simulink model "EPT"  (R2019b)
settings: Solver=FixedStepDiscrete  StartTime=0.0  StopTime=5  FixedStep=0.005  RelTol=1e-3  EnableMultiTasking=on
PreLoadFcn:
  | try, model_open; catch, disp('Error occurred while executing model pre-load callback: model_open.m'); disp('Please assure that the MATLAB working directory is set to the model directory before opening.'); end
InitFcn:
  | try, model_open; catch, end
undefined symbols (not defined in the file or in its folder): Bridge, GCM, H, ln, raptor_get_param_eval, raptor_get_safe_string, raptor_xcp_function
libraries: Raptor_lib x2810, simulink x374, hdlsllib x19
(part 15 of 45)

== system EPT/Foreground_TimeBase_5ms/CAN/CAN2_exec/BCU vs ITRI//ARTC/Remote DAG2-5E1 ==
  Enable : EnablePort
  Trigger : TriggerPort  VariantControl=Variant  PortDimensions=1
  Data Type Conversion{1..4} (4 alike) : DataTypeConversion
  Fcn1 : Fcn  Expr=(u(1)-2)/0.01
  Fcn2 : Fcn  Expr=(u(1)-2)/0.01
  Fcn3 : Fcn  Expr=(u(1)+40)/0.5
  Fcn4 : Fcn  Expr=(u(1)+40)/0.5
  raptor_can_txmsg : Raptor_lib/CAN/raptor_can_txmsg  canDefinition=struct('dbcFile', 'BCUvsRMDA_CMU.dbc','message', 'RemoteDAG_5E1','comment', '','signals', {{'CMU1_Ibp','CMU1_Tcell_Max','CMU1_Tcell_Min','CMU1_Vbp','CMU1_Vcell_Max','CMU1_Vcell_Min'}},'enabled', [ 1 1 1 1 1 1;],'canBus', '''CAN2''','messageID', [ 1505;],'idMask', [ 536870911;],'payloadMask', [],'payloadValue', [],'period', [ 0;],'mailbox', '','queueSize', [ 1;],'label', [ 0;],'ver', [ 2;],'showID', [ 0;],'showRaw', [ 0;],'fill', [ 0;],'editID', [ 0;],'signalOrder', [ 1;])  canBus='CAN2'  queueSize=1  payloadMask=[]  payloadValue=[]  period=0  showID=0  label=0  idMask=hex2dec('1FFFFFFF')  fill=0  id=1505  showRaw=0  signalOrder=1  signalInfo={{struct('Name', 'CMU1_Ibp','Startbit', [ 0;],'SignalSize', [ 16;],'ByteOrder', 'BigEndian','ValueType', 'UNSIGNED','Class', 'uint16','Signed', [ 0;],'Factor', [ 0.02;],'Offset', [ -500;],'Min', [ 0;],'Max', [ 0;],'Units', '','Comment', '','StartBit', [ 8;]),struct('Name', 'CMU1_Vbp','Startbit', [ 0;],'SignalSize', [ 16;],'ByteOrder', 'BigEndian','ValueType', 'UNSIGNED','Class', 'uint16','Signed', [ 0;],'Factor', [ 0.01;],'Offset', [ 0;],'Min', [ 0;],'Max', [ 0;],'Units', '','Comment', '','StartBit', [ 24;]),struct('Name', 'CMU1_Vcell_Max','Startbit', [ 0;],'SignalSize', [ 8;],'ByteOrder', 'BigEndian','ValueType', 'UNSIGNED','Class', 'uint8','Signed', [ 0;],'Factor', [ 1;],'Offset', [ 0;],'Min', [ 0;],'Max', [ 0;],'Units', '','Comment', '','StartBit', [ 32;]),struct('Name', 'CMU1_Vcell_Min','Startbit', [ 0;],'SignalSize', [ 8;],'ByteOrder', 'BigEndian','ValueType', 'UNSIGNED','Class', 'uint8','Signed', [ 0;],'Factor', [ 1;],'Offset', [ 0;],'Min', [ 0;],'Max', [ 0;],'Units', '','Comment', '','StartBit', [ 40;]),struct('Name', 'CMU1_Tcell_Max','Startbit', [ 0;],'SignalSize', [ 8;],'ByteOrder', 'BigEndian','ValueType', 'UNSIGNED','Class', 'uint8','Signed', [ 0;],'Factor', [ 1;],'Offset', [ 0;],'Min', [ 0;],'Max', [ 0;],'Units', '','Comment', '','StartBit', [ 48;]),struct('Name', 'CMU1_Tcell_Min','Startbit', [ 0;],'SignalSize', [ 8;],'ByteOrder', 'BigEndian','ValueType', 'UNSIGNED','Class', 'uint8','Signed', [ 0;],'Factor', [ 1;],'Offset', [ 0;],'Min', [ 0;],'Max', [ 0;],'Units', '','Comment', '','StartBit', [ 56;])}}
      settings: SourceProductName=Raptor
  raptor_data_read : Raptor_lib/Data Storage/raptor_data_read  dataName='CMU1_CELL_VOLT_MAX'  dataShape=Scalar  idxSource=Input  idxRow=1  idxCol=1
      settings: SourceProductName=Raptor
  raptor_data_read1 : Raptor_lib/Data Storage/raptor_data_read  dataName='CMU1_CELL_VOLT_MIN'  dataShape=Scalar  idxSource=Input  idxRow=1  idxCol=1
      settings: SourceProductName=Raptor
  raptor_data_read2 : Raptor_lib/Data Storage/raptor_data_read  dataName='CMU1_CELL_TEMP_MIN'  dataShape=Scalar  idxSource=Input  idxRow=1  idxCol=1
      settings: SourceProductName=Raptor
  raptor_data_read3 : Raptor_lib/Data Storage/raptor_data_read  dataName='CMU1_BATT_CURR'  dataShape=Scalar  idxSource=Input  idxRow=1  idxCol=1
      settings: SourceProductName=Raptor
  raptor_data_read4 : Raptor_lib/Data Storage/raptor_data_read  dataName='CMU1_BATT_VOLT'  dataShape=Scalar  idxSource=Input  idxRow=1  idxCol=1
      settings: SourceProductName=Raptor
  raptor_data_read5 : Raptor_lib/Data Storage/raptor_data_read  dataName='CMU1_CELL_TEMP_MAX'  dataShape=Scalar  idxSource=Input  idxRow=1  idxCol=1
      settings: SourceProductName=Raptor
  wires:
  Fcn4/1 -> Data Type Conversion3/1
  Data Type Conversion3/1 -> raptor_can_txmsg/3
  raptor_data_read2/1 -> Fcn4/1
  raptor_data_read5/1 -> Fcn3/1
  Data Type Conversion2/1 -> raptor_can_txmsg/2
  Fcn3/1 -> Data Type Conversion2/1
  Data Type Conversion1/1 -> raptor_can_txmsg/5
  Data Type Conversion4/1 -> raptor_can_txmsg/6
  Fcn1/1 -> Data Type Conversion4/1
  Fcn2/1 -> Data Type Conversion1/1
  raptor_data_read4/1 -> raptor_can_txmsg/4
  raptor_data_read3/1 -> raptor_can_txmsg/1
  raptor_data_read1/1 -> Fcn1/1
  raptor_data_read/1 -> Fcn2/1

== system EPT/Foreground_TimeBase_5ms/CAN/CAN2_exec/BCU vs ITRI//ARTC/Remote DAG2-5E2 ==
  Enable : EnablePort
  Trigger : TriggerPort  VariantControl=Variant  PortDimensions=1
  Data Type Conversion{1..8} (8 alike) : DataTypeConversion
  Fcn{,1..7} (8 alike) : Fcn  Expr=(u(1)-2)/0.01
  raptor_can_txmsg : Raptor_lib/CAN/raptor_can_txmsg  canDefinition=struct('dbcFile', 'BCUvsRMDA_CMU.dbc','message', 'RemoteDAG_5E2','comment', '','signals', {{'CMU1_Vcell_V01','CMU1_Vcell_V02','CMU1_Vcell_V03','CMU1_Vcell_V04','CMU1_Vcell_V05','CMU1_Vcell_V06','CMU1_Vcell_V07','CMU1_Vcell_V08'}},'enabled', [ 1 1 1 1 1 1 1 1;],'canBus', '''CAN2''','messageID', [ 1506;],'idMask', [ 536870911;],'payloadMask', [],'payloadValue', [],'period', [ 0;],'mailbox', '','queueSize', [ 1;],'label', [ 0;],'ver', [ 2;],'showID', [ 0;],'showRaw', [ 0;],'fill', [ 0;],'editID', [ 0;],'signalOrder', [ 1;])  canBus='CAN2'  queueSize=1  payloadMask=[]  payloadValue=[]  period=0  showID=0  label=0  idMask=hex2dec('1FFFFFFF')  fill=0  id=1506  showRaw=0  signalOrder=1  signalInfo={{struct('Name', 'CMU1_Vcell_V01','Startbit', [ 0;],'SignalSize', [ 8;],'ByteOrder', 'BigEndian','ValueType', 'UNSIGNED','Class', 'uint8','Signed', [ 0;],'Factor', [ 1;],'Offset', [ 0;],'Min', [ 0;],'Max', [ 0;],'Units', '','Comment', '','StartBit', [ 0;]),struct('Name', 'CMU1_Vcell_V02','Startbit', [ 0;],'SignalSize', [ 8;],'ByteOrder', 'BigEndian','ValueType', 'UNSIGNED','Class', 'uint8','Signed', [ 0;],'Factor', [ 1;],'Offset', [ 0;],'Min', [ 0;],'Max', [ 0;],'Units', '','Comment', '','StartBit', [ 8;]),struct('Name', 'CMU1_Vcell_V03','Startbit', [ 0;],'SignalSize', [ 8;],'ByteOrder', 'BigEndian','ValueType', 'UNSIGNED','Class', 'uint8','Signed', [ 0;],'Factor', [ 1;],'Offset', [ 0;],'Min', [ 0;],'Max', [ 0;],'Units', '','Comment', '','StartBit', [ 16;]),struct('Name', 'CMU1_Vcell_V04','Startbit', [ 0;],'SignalSize', [ 8;],'ByteOrder', 'BigEndian','ValueType', 'UNSIGNED','Class', 'uint8','Signed', [ 0;],'Factor', [ 1;],'Offset', [ 0;],'Min', [ 0;],'Max', [ 0;],'Units', '','Comment', '','StartBit', [ 24;]),struct('Name', 'CMU1_Vcell_V05','Startbit', [ 0;],'SignalSize', [ 8;],'ByteOrder', 'BigEndian','ValueType', 'UNSIGNED','Class', 'uint8','Signed', [ 0;],'Factor', [ 1;],'Offset', [ 0;],'Min', [ 0;],'Max', [ 0;],'Units', '','Comment', '','StartBit', [ 32;]),struct('Name', 'CMU1_Vcell_V06','Startbit', [ 0;],'SignalSize', [ 8;],'ByteOrder', 'BigEndian','ValueType', 'UNSIGNED','Class', 'uint8','Signed', [ 0;],'Factor', [ 1;],'Offset', [ 0;],'Min', [ 0;],'Max', [ 0;],'Units', '','Comment', '','StartBit', [ 40;]),struct('Name', 'CMU1_Vcell_V07','Startbit', [ 0;],'SignalSize', [ 8;],'ByteOrder', 'BigEndian','ValueType', 'UNSIGNED','Class', 'uint8','Signed', [ 0;],'Factor', [ 1;],'Offset', [ 0;],'Min', [ 0;],'Max', [ 0;],'Units', '','Comment', '','StartBit', [ 48;]),struct('Name', 'CMU1_Vcell_V08','Startbit', [ 0;],'SignalSize', [ 8;],'ByteOrder', 'BigEndian','ValueType', 'UNSIGNED','Class', 'uint8','Signed', [ 0;],'Factor', [ 1;],'Offset', [ 0;],'Min', [ 0;],'Max', [ 0;],'Units', '','Comment', '','StartBit', [ 56;])}}
      settings: SourceProductName=Raptor
  raptor_data_read1 : Raptor_lib/Data Storage/raptor_data_read  dataName='CMU1_CELL02_VOLT'  dataShape=Scalar  idxSource=Input  idxRow=1  idxCol=1
      settings: SourceProductName=Raptor
  raptor_data_read2 : Raptor_lib/Data Storage/raptor_data_read  dataName='CMU1_CELL03_VOLT'  dataShape=Scalar  idxSource=Input  idxRow=1  idxCol=1
      settings: SourceProductName=Raptor
  raptor_data_read3 : Raptor_lib/Data Storage/raptor_data_read  dataName='CMU1_CELL01_VOLT'  dataShape=Scalar  idxSource=Input  idxRow=1  idxCol=1
      settings: SourceProductName=Raptor
  raptor_data_read4 : Raptor_lib/Data Storage/raptor_data_read  dataName='CMU1_CELL04_VOLT'  dataShape=Scalar  idxSource=Input  idxRow=1  idxCol=1
      settings: SourceProductName=Raptor
  raptor_data_read5 : Raptor_lib/Data Storage/raptor_data_read  dataName='CMU1_CELL05_VOLT'  dataShape=Scalar  idxSource=Input  idxRow=1  idxCol=1
      settings: SourceProductName=Raptor
  raptor_data_read6 : Raptor_lib/Data Storage/raptor_data_read  dataName='CMU1_CELL06_VOLT'  dataShape=Scalar  idxSource=Input  idxRow=1  idxCol=1
      settings: SourceProductName=Raptor
  raptor_data_read7 : Raptor_lib/Data Storage/raptor_data_read  dataName='CMU1_CELL07_VOLT'  dataShape=Scalar  idxSource=Input  idxRow=1  idxCol=1
      settings: SourceProductName=Raptor
  raptor_data_read8 : Raptor_lib/Data Storage/raptor_data_read  dataName='CMU1_CELL08_VOLT'  dataShape=Scalar  idxSource=Input  idxRow=1  idxCol=1
      settings: SourceProductName=Raptor
  wires:
  raptor_data_read7/1 -> Fcn6/1
  raptor_data_read6/1 -> Fcn5/1
  raptor_data_read5/1 -> Fcn4/1
  raptor_data_read4/1 -> Fcn3/1
  raptor_data_read2/1 -> Fcn2/1
  raptor_data_read3/1 -> Fcn/1
  Data Type Conversion4/1 -> raptor_can_txmsg/1
  Fcn1/1 -> Data Type Conversion8/1
  Fcn2/1 -> Data Type Conversion7/1
  Fcn7/1 -> Data Type Conversion3/1
  Data Type Conversion2/1 -> raptor_can_txmsg/7
  Data Type Conversion8/1 -> raptor_can_txmsg/2
  Data Type Conversion1/1 -> raptor_can_txmsg/6
  Data Type Conversion5/1 -> raptor_can_txmsg/5
  Data Type Conversion6/1 -> raptor_can_txmsg/4
  Data Type Conversion7/1 -> raptor_can_txmsg/3
  Data Type Conversion3/1 -> raptor_can_txmsg/8
  Fcn3/1 -> Data Type Conversion6/1
  Fcn4/1 -> Data Type Conversion5/1
  Fcn6/1 -> Data Type Conversion2/1
  Fcn/1 -> Data Type Conversion4/1
  Fcn5/1 -> Data Type Conversion1/1
  raptor_data_read8/1 -> Fcn7/1
  raptor_data_read1/1 -> Fcn1/1

== system EPT/Foreground_TimeBase_5ms/CAN/CAN2_exec/BCU vs ITRI//ARTC/Remote DAG2-5E3 ==
  Enable : EnablePort
  Trigger : TriggerPort  VariantControl=Variant  PortDimensions=1
  Data Type Conversion{1..8} (8 alike) : DataTypeConversion
  Fcn{,1..7} (8 alike) : Fcn  Expr=(u(1)-2)/0.01
  raptor_can_txmsg : Raptor_lib/CAN/raptor_can_txmsg  canDefinition=struct('dbcFile', 'BCUvsRMDA_CMU.dbc','message', 'RemoteDAG_5E3','comment', '','signals', {{'CMU1_Vcell_V09','CMU1_Vcell_V10','CMU1_Vcell_V11','CMU1_Vcell_V12','CMU1_Vcell_V13','CMU1_Vcell_V14','CMU1_Vcell_V15','CMU1_Vcell_V16'}},'enabled', [ 1 1 1 1 1 1 1 1;],'canBus', '''CAN2''','messageID', [ 1507;],'idMask', [ 536870911;],'payloadMask', [],'payloadValue', [],'period', [ 0;],'mailbox', '','queueSize', [ 1;],'label', [ 0;],'ver', [ 2;],'showID', [ 0;],'showRaw', [ 0;],'fill', [ 0;],'editID', [ 0;],'signalOrder', [ 1;])  canBus='CAN2'  queueSize=1  payloadMask=[]  payloadValue=[]  period=0  showID=0  label=0  idMask=hex2dec('1FFFFFFF')  fill=0  id=1507  showRaw=0  signalOrder=1  signalInfo={{struct('Name', 'CMU1_Vcell_V09','Startbit', [ 0;],'SignalSize', [ 8;],'ByteOrder', 'BigEndian','ValueType', 'UNSIGNED','Class', 'uint8','Signed', [ 0;],'Factor', [ 1;],'Offset', [ 0;],'Min', [ 0;],'Max', [ 0;],'Units', '','Comment', '','StartBit', [ 0;]),struct('Name', 'CMU1_Vcell_V10','Startbit', [ 0;],'SignalSize', [ 8;],'ByteOrder', 'BigEndian','ValueType', 'UNSIGNED','Class', 'uint8','Signed', [ 0;],'Factor', [ 1;],'Offset', [ 0;],'Min', [ 0;],'Max', [ 0;],'Units', '','Comment', '','StartBit', [ 8;]),struct('Name', 'CMU1_Vcell_V11','Startbit', [ 0;],'SignalSize', [ 8;],'ByteOrder', 'BigEndian','ValueType', 'UNSIGNED','Class', 'uint8','Signed', [ 0;],'Factor', [ 1;],'Offset', [ 0;],'Min', [ 0;],'Max', [ 0;],'Units', '','Comment', '','StartBit', [ 16;]),struct('Name', 'CMU1_Vcell_V12','Startbit', [ 0;],'SignalSize', [ 8;],'ByteOrder', 'BigEndian','ValueType', 'UNSIGNED','Class', 'uint8','Signed', [ 0;],'Factor', [ 1;],'Offset', [ 0;],'Min', [ 0;],'Max', [ 0;],'Units', '','Comment', '','StartBit', [ 24;]),struct('Name', 'CMU1_Vcell_V13','Startbit', [ 0;],'SignalSize', [ 8;],'ByteOrder', 'BigEndian','ValueType', 'UNSIGNED','Class', 'uint8','Signed', [ 0;],'Factor', [ 1;],'Offset', [ 0;],'Min', [ 0;],'Max', [ 0;],'Units', '','Comment', '','StartBit', [ 32;]),struct('Name', 'CMU1_Vcell_V14','Startbit', [ 0;],'SignalSize', [ 8;],'ByteOrder', 'BigEndian','ValueType', 'UNSIGNED','Class', 'uint8','Signed', [ 0;],'Factor', [ 1;],'Offset', [ 0;],'Min', [ 0;],'Max', [ 0;],'Units', '','Comment', '','StartBit', [ 40;]),struct('Name', 'CMU1_Vcell_V15','Startbit', [ 0;],'SignalSize', [ 8;],'ByteOrder', 'BigEndian','ValueType', 'UNSIGNED','Class', 'uint8','Signed', [ 0;],'Factor', [ 1;],'Offset', [ 0;],'Min', [ 0;],'Max', [ 0;],'Units', '','Comment', '','StartBit', [ 48;]),struct('Name', 'CMU1_Vcell_V16','Startbit', [ 0;],'SignalSize', [ 8;],'ByteOrder', 'BigEndian','ValueType', 'UNSIGNED','Class', 'uint8','Signed', [ 0;],'Factor', [ 1;],'Offset', [ 0;],'Min', [ 0;],'Max', [ 0;],'Units', '','Comment', '','StartBit', [ 56;])}}
      settings: SourceProductName=Raptor
  raptor_data_read1 : Raptor_lib/Data Storage/raptor_data_read  dataName='CMU1_CELL10_VOLT'  dataShape=Scalar  idxSource=Input  idxRow=1  idxCol=1
      settings: SourceProductName=Raptor
  raptor_data_read2 : Raptor_lib/Data Storage/raptor_data_read  dataName='CMU1_CELL11_VOLT'  dataShape=Scalar  idxSource=Input  idxRow=1  idxCol=1
      settings: SourceProductName=Raptor
  raptor_data_read3 : Raptor_lib/Data Storage/raptor_data_read  dataName='CMU1_CELL09_VOLT'  dataShape=Scalar  idxSource=Input  idxRow=1  idxCol=1
      settings: SourceProductName=Raptor
  raptor_data_read4 : Raptor_lib/Data Storage/raptor_data_read  dataName='CMU1_CELL12_VOLT'  dataShape=Scalar  idxSource=Input  idxRow=1  idxCol=1
      settings: SourceProductName=Raptor
  raptor_data_read5 : Raptor_lib/Data Storage/raptor_data_read  dataName='CMU1_CELL13_VOLT'  dataShape=Scalar  idxSource=Input  idxRow=1  idxCol=1
      settings: SourceProductName=Raptor
  raptor_data_read6 : Raptor_lib/Data Storage/raptor_data_read  dataName='CMU1_CELL14_VOLT'  dataShape=Scalar  idxSource=Input  idxRow=1  idxCol=1
      settings: SourceProductName=Raptor
  raptor_data_read7 : Raptor_lib/Data Storage/raptor_data_read  dataName='CMU1_CELL15_VOLT'  dataShape=Scalar  idxSource=Input  idxRow=1  idxCol=1
      settings: SourceProductName=Raptor
  raptor_data_read8 : Raptor_lib/Data Storage/raptor_data_read  dataName='CMU1_CELL16_VOLT'  dataShape=Scalar  idxSource=Input  idxRow=1  idxCol=1
      settings: SourceProductName=Raptor
  wires:
  Fcn7/1 -> Data Type Conversion3/1
  Fcn6/1 -> Data Type Conversion2/1
  Fcn5/1 -> Data Type Conversion1/1
  Fcn4/1 -> Data Type Conversion5/1
  Fcn3/1 -> Data Type Conversion6/1
  Fcn2/1 -> Data Type Conversion7/1
  Fcn1/1 -> Data Type Conversion8/1
  Fcn/1 -> Data Type Conversion4/1
  raptor_data_read8/1 -> Fcn7/1
  raptor_data_read7/1 -> Fcn6/1
  raptor_data_read6/1 -> Fcn5/1
  raptor_data_read3/1 -> Fcn/1
  raptor_data_read4/1 -> Fcn3/1
  raptor_data_read2/1 -> Fcn2/1
  raptor_data_read1/1 -> Fcn1/1
  Data Type Conversion5/1 -> raptor_can_txmsg/5
  raptor_data_read5/1 -> Fcn4/1
  Data Type Conversion3/1 -> raptor_can_txmsg/8
  Data Type Conversion2/1 -> raptor_can_txmsg/7
  Data Type Conversion1/1 -> raptor_can_txmsg/6
  Data Type Conversion6/1 -> raptor_can_txmsg/4
  Data Type Conversion7/1 -> raptor_can_txmsg/3
  Data Type Conversion8/1 -> raptor_can_txmsg/2
  Data Type Conversion4/1 -> raptor_can_txmsg/1

== system EPT/Foreground_TimeBase_5ms/CAN/CAN2_exec/BCU vs ITRI//ARTC/Remote DAG2-5E4 ==
  Enable : EnablePort
  Trigger : TriggerPort  VariantControl=Variant  PortDimensions=1
  Data Type Conversion{1..8} (8 alike) : DataTypeConversion
  Fcn{1..8} (8 alike) : Fcn  Expr=(u(1)+40)/0.5
  raptor_can_txmsg : Raptor_lib/CAN/raptor_can_txmsg  canDefinition=struct('dbcFile', 'BCUvsRMDA_CMU.dbc','message', 'RemoteDAG_5E4','comment', '','signals', {{'CMU1_Tcell_T01','CMU1_Tcell_T02','CMU1_Tcell_T03','CMU1_Tcell_T04','CMU1_Tcell_T05','CMU1_Tcell_T06','CMU1_Tcell_T07','CMU1_Tcell_T08'}},'enabled', [ 1 1 1 1 1 1 1 1;],'canBus', '''CAN2''','messageID', [ 1508;],'idMask', [ 536870911;],'payloadMask', [],'payloadValue', [],'period', [ 0;],'mailbox', '','queueSize', [ 1;],'label', [ 0;],'ver', [ 2;],'showID', [ 0;],'showRaw', [ 0;],'fill', [ 0;],'editID', [ 0;],'signalOrder', [ 1;])  canBus='CAN2'  queueSize=1  payloadMask=[]  payloadValue=[]  period=0  showID=0  label=0  idMask=hex2dec('1FFFFFFF')  fill=0  id=1508  showRaw=0  signalOrder=1  signalInfo={{struct('Name', 'CMU1_Tcell_T01','Startbit', [ 0;],'SignalSize', [ 8;],'ByteOrder', 'BigEndian','ValueType', 'UNSIGNED','Class', 'uint8','Signed', [ 0;],'Factor', [ 1;],'Offset', [ 0;],'Min', [ 0;],'Max', [ 0;],'Units', '','Comment', '','StartBit', [ 0;]),struct('Name', 'CMU1_Tcell_T02','Startbit', [ 0;],'SignalSize', [ 8;],'ByteOrder', 'BigEndian','ValueType', 'UNSIGNED','Class', 'uint8','Signed', [ 0;],'Factor', [ 1;],'Offset', [ 0;],'Min', [ 0;],'Max', [ 0;],'Units', '','Comment', '','StartBit', [ 8;]),struct('Name', 'CMU1_Tcell_T03','Startbit', [ 0;],'SignalSize', [ 8;],'ByteOrder', 'BigEndian','ValueType', 'UNSIGNED','Class', 'uint8','Signed', [ 0;],'Factor', [ 1;],'Offset', [ 0;],'Min', [ 0;],'Max', [ 0;],'Units', '','Comment', '','StartBit', [ 16;]),struct('Name', 'CMU1_Tcell_T04','Startbit', [ 0;],'SignalSize', [ 8;],'ByteOrder', 'BigEndian','ValueType', 'UNSIGNED','Class', 'uint8','Signed', [ 0;],'Factor', [ 1;],'Offset', [ 0;],'Min', [ 0;],'Max', [ 0;],'Units', '','Comment', '','StartBit', [ 24;]),struct('Name', 'CMU1_Tcell_T05','Startbit', [ 0;],'SignalSize', [ 8;],'ByteOrder', 'BigEndian','ValueType', 'UNSIGNED','Class', 'uint8','Signed', [ 0;],'Factor', [ 1;],'Offset', [ 0;],'Min', [ 0;],'Max', [ 0;],'Units', '','Comment', '','StartBit', [ 32;]),struct('Name', 'CMU1_Tcell_T06','Startbit', [ 0;],'SignalSize', [ 8;],'ByteOrder', 'BigEndian','ValueType', 'UNSIGNED','Class', 'uint8','Signed', [ 0;],'Factor', [ 1;],'Offset', [ 0;],'Min', [ 0;],'Max', [ 0;],'Units', '','Comment', '','StartBit', [ 40;]),struct('Name', 'CMU1_Tcell_T07','Startbit', [ 0;],'SignalSize', [ 8;],'ByteOrder', 'BigEndian','ValueType', 'UNSIGNED','Class', 'uint8','Signed', [ 0;],'Factor', [ 1;],'Offset', [ 0;],'Min', [ 0;],'Max', [ 0;],'Units', '','Comment', '','StartBit', [ 48;]),struct('Name', 'CMU1_Tcell_T08','Startbit', [ 0;],'SignalSize', [ 8;],'ByteOrder', 'BigEndian','ValueType', 'UNSIGNED','Class', 'uint8','Signed', [ 0;],'Factor', [ 1;],'Offset', [ 0;],'Min', [ 0;],'Max', [ 0;],'Units', '','Comment', '','StartBit', [ 56;])}}
      settings: SourceProductName=Raptor
  raptor_data_read1 : Raptor_lib/Data Storage/raptor_data_read  dataName='CMU1_CELL02_TEMP'  dataShape=Scalar  idxSource=Input  idxRow=1  idxCol=1
      settings: SourceProductName=Raptor
  raptor_data_read2 : Raptor_lib/Data Storage/raptor_data_read  dataName='CMU1_CELL03_TEMP'  dataShape=Scalar  idxSource=Input  idxRow=1  idxCol=1
      settings: SourceProductName=Raptor
  raptor_data_read3 : Raptor_lib/Data Storage/raptor_data_read  dataName='CMU1_CELL01_TEMP'  dataShape=Scalar  idxSource=Input  idxRow=1  idxCol=1
      settings: SourceProductName=Raptor
  raptor_data_read4 : Raptor_lib/Data Storage/raptor_data_read  dataName='CMU1_CELL04_TEMP'  dataShape=Scalar  idxSource=Input  idxRow=1  idxCol=1
      settings: SourceProductName=Raptor
  raptor_data_read5 : Raptor_lib/Data Storage/raptor_data_read  dataName='CMU1_CELL05_TEMP'  dataShape=Scalar  idxSource=Input  idxRow=1  idxCol=1
      settings: SourceProductName=Raptor
  raptor_data_read6 : Raptor_lib/Data Storage/raptor_data_read  dataName='CMU1_CELL06_TEMP'  dataShape=Scalar  idxSource=Input  idxRow=1  idxCol=1
      settings: SourceProductName=Raptor
  raptor_data_read7 : Raptor_lib/Data Storage/raptor_data_read  dataName='CMU1_CELL07_TEMP'  dataShape=Scalar  idxSource=Input  idxRow=1  idxCol=1
      settings: SourceProductName=Raptor
  raptor_data_read8 : Raptor_lib/Data Storage/raptor_data_read  dataName='CMU1_CELL08_TEMP'  dataShape=Scalar  idxSource=Input  idxRow=1  idxCol=1
      settings: SourceProductName=Raptor
  wires:
  Data Type Conversion8/1 -> raptor_can_txmsg/8
  Data Type Conversion7/1 -> raptor_can_txmsg/7
  Data Type Conversion6/1 -> raptor_can_txmsg/6
  Data Type Conversion5/1 -> raptor_can_txmsg/5
  Data Type Conversion4/1 -> raptor_can_txmsg/4
  Data Type Conversion2/1 -> raptor_can_txmsg/3
  Data Type Conversion1/1 -> raptor_can_txmsg/2
  Data Type Conversion3/1 -> raptor_can_txmsg/1
  Fcn8/1 -> Data Type Conversion8/1
  Fcn7/1 -> Data Type Conversion7/1
  Fcn6/1 -> Data Type Conversion6/1
  Fcn5/1 -> Data Type Conversion5/1
  Fcn4/1 -> Data Type Conversion4/1
  Fcn3/1 -> Data Type Conversion2/1
  Fcn1/1 -> Data Type Conversion1/1
  Fcn2/1 -> Data Type Conversion3/1
  raptor_data_read8/1 -> Fcn8/1
  raptor_data_read7/1 -> Fcn7/1
  raptor_data_read6/1 -> Fcn6/1
  raptor_data_read5/1 -> Fcn5/1
  raptor_data_read3/1 -> Fcn2/1
  raptor_data_read1/1 -> Fcn1/1
  raptor_data_read2/1 -> Fcn3/1
  raptor_data_read4/1 -> Fcn4/1

== system EPT/Foreground_TimeBase_5ms/CAN/CAN2_exec/BCU vs ITRI//ARTC/Remote DAG2-5E5 ==
  Enable : EnablePort
  Trigger : TriggerPort  VariantControl=Variant  PortDimensions=1
  Data Type Conversion{1..8} (8 alike) : DataTypeConversion
  Fcn{1..8} (8 alike) : Fcn  Expr=(u(1)+40)/0.5
  raptor_can_txmsg : Raptor_lib/CAN/raptor_can_txmsg  canDefinition=struct('dbcFile', 'BCUvsRMDA_CMU.dbc','message', 'RemoteDAG_5E5','comment', '','signals', {{'CMU1_Tcell_T09','CMU1_Tcell_T10','CMU1_Tcell_T11','CMU1_Tcell_T12','CMU1_Tcell_T13','CMU1_Tcell_T14','CMU1_Tcell_T15','CMU1_Tcell_T16'}},'enabled', [ 1 1 1 1 1 1 1 1;],'canBus', '''CAN2''','messageID', [ 1509;],'idMask', [ 536870911;],'payloadMask', [],'payloadValue', [],'period', [ 0;],'mailbox', '','queueSize', [ 1;],'label', [ 0;],'ver', [ 2;],'showID', [ 0;],'showRaw', [ 0;],'fill', [ 0;],'editID', [ 0;],'signalOrder', [ 1;])  canBus='CAN2'  queueSize=1  payloadMask=[]  payloadValue=[]  period=0  showID=0  label=0  idMask=hex2dec('1FFFFFFF')  fill=0  id=1509  showRaw=0  signalOrder=1  signalInfo={{struct('Name', 'CMU1_Tcell_T09','Startbit', [ 0;],'SignalSize', [ 8;],'ByteOrder', 'BigEndian','ValueType', 'UNSIGNED','Class', 'uint8','Signed', [ 0;],'Factor', [ 1;],'Offset', [ 0;],'Min', [ 0;],'Max', [ 0;],'Units', '','Comment', '','StartBit', [ 0;]),struct('Name', 'CMU1_Tcell_T10','Startbit', [ 0;],'SignalSize', [ 8;],'ByteOrder', 'BigEndian','ValueType', 'UNSIGNED','Class', 'uint8','Signed', [ 0;],'Factor', [ 1;],'Offset', [ 0;],'Min', [ 0;],'Max', [ 0;],'Units', '','Comment', '','StartBit', [ 8;]),struct('Name', 'CMU1_Tcell_T11','Startbit', [ 0;],'SignalSize', [ 8;],'ByteOrder', 'BigEndian','ValueType', 'UNSIGNED','Class', 'uint8','Signed', [ 0;],'Factor', [ 1;],'Offset', [ 0;],'Min', [ 0;],'Max', [ 0;],'Units', '','Comment', '','StartBit', [ 16;]),struct('Name', 'CMU1_Tcell_T12','Startbit', [ 0;],'SignalSize', [ 8;],'ByteOrder', 'BigEndian','ValueType', 'UNSIGNED','Class', 'uint8','Signed', [ 0;],'Factor', [ 1;],'Offset', [ 0;],'Min', [ 0;],'Max', [ 0;],'Units', '','Comment', '','StartBit', [ 24;]),struct('Name', 'CMU1_Tcell_T13','Startbit', [ 0;],'SignalSize', [ 8;],'ByteOrder', 'BigEndian','ValueType', 'UNSIGNED','Class', 'uint8','Signed', [ 0;],'Factor', [ 1;],'Offset', [ 0;],'Min', [ 0;],'Max', [ 0;],'Units', '','Comment', '','StartBit', [ 32;]),struct('Name', 'CMU1_Tcell_T14','Startbit', [ 0;],'SignalSize', [ 8;],'ByteOrder', 'BigEndian','ValueType', 'UNSIGNED','Class', 'uint8','Signed', [ 0;],'Factor', [ 1;],'Offset', [ 0;],'Min', [ 0;],'Max', [ 0;],'Units', '','Comment', '','StartBit', [ 40;]),struct('Name', 'CMU1_Tcell_T15','Startbit', [ 0;],'SignalSize', [ 8;],'ByteOrder', 'BigEndian','ValueType', 'UNSIGNED','Class', 'uint8','Signed', [ 0;],'Factor', [ 1;],'Offset', [ 0;],'Min', [ 0;],'Max', [ 0;],'Units', '','Comment', '','StartBit', [ 48;]),struct('Name', 'CMU1_Tcell_T16','Startbit', [ 0;],'SignalSize', [ 8;],'ByteOrder', 'BigEndian','ValueType', 'UNSIGNED','Class', 'uint8','Signed', [ 0;],'Factor', [ 1;],'Offset', [ 0;],'Min', [ 0;],'Max', [ 0;],'Units', '','Comment', '','StartBit', [ 56;])}}
      settings: SourceProductName=Raptor
  raptor_data_read1 : Raptor_lib/Data Storage/raptor_data_read  dataName='CMU1_CELL11_TEMP'  dataShape=Scalar  idxSource=Input  idxRow=1  idxCol=1
      settings: SourceProductName=Raptor
  raptor_data_read2 : Raptor_lib/Data Storage/raptor_data_read  dataName='CMU1_CELL09_TEMP'  dataShape=Scalar  idxSource=Input  idxRow=1  idxCol=1
      settings: SourceProductName=Raptor
  raptor_data_read3 : Raptor_lib/Data Storage/raptor_data_read  dataName='CMU1_CELL10_TEMP'  dataShape=Scalar  idxSource=Input  idxRow=1  idxCol=1
      settings: SourceProductName=Raptor
  raptor_data_read4 : Raptor_lib/Data Storage/raptor_data_read  dataName='CMU1_CELL13_TEMP'  dataShape=Scalar  idxSource=Input  idxRow=1  idxCol=1
      settings: SourceProductName=Raptor
  raptor_data_read5 : Raptor_lib/Data Storage/raptor_data_read  dataName='CMU1_CELL12_TEMP'  dataShape=Scalar  idxSource=Input  idxRow=1  idxCol=1
      settings: SourceProductName=Raptor
  raptor_data_read6 : Raptor_lib/Data Storage/raptor_data_read  dataName='CMU1_CELL15_TEMP'  dataShape=Scalar  idxSource=Input  idxRow=1  idxCol=1
      settings: SourceProductName=Raptor
  raptor_data_read7 : Raptor_lib/Data Storage/raptor_data_read  dataName='CMU1_CELL14_TEMP'  dataShape=Scalar  idxSource=Input  idxRow=1  idxCol=1
      settings: SourceProductName=Raptor
  raptor_data_read9 : Raptor_lib/Data Storage/raptor_data_read  dataName='CMU1_CELL16_TEMP'  dataShape=Scalar  idxSource=Input  idxRow=1  idxCol=1
      settings: SourceProductName=Raptor
  wires:
  Fcn3/1 -> Data Type Conversion2/1
  Fcn7/1 -> Data Type Conversion7/1
  Fcn5/1 -> Data Type Conversion5/1
  Data Type Conversion5/1 -> raptor_can_txmsg/5
  Data Type Conversion3/1 -> raptor_can_txmsg/1
  Fcn4/1 -> Data Type Conversion4/1
  Fcn6/1 -> Data Type Conversion6/1
  Fcn1/1 -> Data Type Conversion1/1
  Fcn8/1 -> Data Type Conversion8/1
  Fcn2/1 -> Data Type Conversion3/1
  raptor_data_read1/1 -> Fcn3/1
  Data Type Conversion1/1 -> raptor_can_txmsg/2
  raptor_data_read5/1 -> Fcn4/1
  raptor_data_read3/1 -> Fcn1/1
  raptor_data_read6/1 -> Fcn7/1
  raptor_data_read7/1 -> Fcn6/1
  raptor_data_read9/1 -> Fcn8/1
  raptor_data_read4/1 -> Fcn5/1
  Data Type Conversion6/1 -> raptor_can_txmsg/6
  Data Type Conversion2/1 -> raptor_can_txmsg/3
  raptor_data_read2/1 -> Fcn2/1
  Data Type Conversion4/1 -> raptor_can_txmsg/4
  Data Type Conversion7/1 -> raptor_can_txmsg/7
  Data Type Conversion8/1 -> raptor_can_txmsg/8

== system EPT/Foreground_TimeBase_5ms/CAN/CAN2_exec/BCU vs ITRI//ARTC/Remote DAG2-5E6 ==
  Enable : EnablePort
  Trigger : TriggerPort  VariantControl=Variant  PortDimensions=1
  Bitwise Operator : simulink/Logic and Bit Operations/Bitwise Operator  logicop=AND  UseBitMask=on  BitMask=hex2dec('f0')  BitMaskRealWorld=Stored Integer
  Bitwise Operator1 : simulink/Logic and Bit Operations/Bitwise Operator  logicop=AND  UseBitMask=on  BitMask=hex2dec('0f')  BitMaskRealWorld=Stored Integer
  Data Type Conversion{,1..5} (6 alike) : DataTypeConversion
  Fcn1 : Fcn  Expr=(u(1)+12.5)/0.5
  Shift Arithmetic1 : ArithShift  BitShiftNumber=4  BitShiftDirection=Right
  raptor_can_txmsg : Raptor_lib/CAN/raptor_can_txmsg  canDefinition=struct('dbcFile', 'BCUvsRMDA_CMU.dbc','message', 'RemoteDAG_5E6','comment', '','signals', {{'CMU2_EW_Level3_Hbyte','CMU2_EW_Level3_Lbyte','CMU2_FCC','CMU2_Mode','CMU2_RSOC','CMU2_Rcap'}},'enabled', [ 1 1 1 1 1 1;],'canBus', '''CAN2''','messageID', [ 1510;],'idMask', [ 536870911;],'payloadMask', [],'payloadValue', [],'period', [ 0;],'mailbox', '','queueSize', [ 1;],'label', [ 0;],'ver', [ 2;],'showID', [ 0;],'showRaw', [ 0;],'fill', [ 0;],'editID', [ 0;],'signalOrder', [ 1;])  canBus='CAN2'  queueSize=1  payloadMask=[]  payloadValue=[]  period=0  showID=0  label=0  idMask=hex2dec('1FFFFFFF')  fill=0  id=1510  showRaw=0  signalOrder=1  signalInfo={{struct('Name', 'CMU2_Mode','Startbit', [ 0;],'SignalSize', [ 8;],'ByteOrder', 'BigEndian','ValueType', 'UNSIGNED','Class', 'uint8','Signed', [ 0;],'Factor', [ 1;],'Offset', [ 0;],'Min', [ 0;],'Max', [ 0;],'Units', '','Comment', '','StartBit', [ 0;]),struct('Name', 'CMU2_EW_Level3_Hbyte','Startbit', [ 0;],'SignalSize', [ 8;],'ByteOrder', 'BigEndian','ValueType', 'UNSIGNED','Class', 'uint8','Signed', [ 0;],'Factor', [ 1;],'Offset', [ 0;],'Min', [ 0;],'Max', [ 0;],'Units', '','Comment', '','StartBit', [ 8;]),struct('Name', 'CMU2_EW_Level3_Lbyte','Startbit', [ 0;],'SignalSize', [ 8;],'ByteOrder', 'BigEndian','ValueType', 'UNSIGNED','Class', 'uint8','Signed', [ 0;],'Factor', [ 1;],'Offset', [ 0;],'Min', [ 0;],'Max', [ 0;],'Units', '','Comment', '','StartBit', [ 16;]),struct('Name', 'CMU2_FCC','Startbit', [ 0;],'SignalSize', [ 8;],'ByteOrder', 'BigEndian','ValueType', 'UNSIGNED','Class', 'uint8','Signed', [ 0;],'Factor', [ 1;],'Offset', [ 0;],'Min', [ 0;],'Max', [ 0;],'Units', '','Comment', '','StartBit', [ 32;]),struct('Name', 'CMU2_Rcap','Startbit', [ 0;],'SignalSize', [ 8;],'ByteOrder', 'BigEndian','ValueType', 'UNSIGNED','Class', 'uint8','Signed', [ 0;],'Factor', [ 1;],'Offset', [ 0;],'Min', [ 0;],'Max', [ 0;],'Units', '','Comment', '','StartBit', [ 40;]),struct('Name', 'CMU2_RSOC','Startbit', [ 0;],'SignalSize', [ 8;],'ByteOrder', 'BigEndian','ValueType', 'UNSIGNED','Class', 'uint8','Signed', [ 0;],'Factor', [ 1;],'Offset', [ 0;],'Min', [ 0;],'Max', [ 0;],'Units', '','Comment', '','StartBit', [ 48;])}}
      settings: SourceProductName=Raptor
  raptor_data_read1 : Raptor_lib/Data Storage/raptor_data_read  dataName='CMU2_RSOC'  dataShape=Scalar  idxSource=Input  idxRow=1  idxCol=1
      settings: SourceProductName=Raptor
  raptor_data_read2 : Raptor_lib/Data Storage/raptor_data_read  dataName='CMU2_STATUS'  dataShape=Scalar  idxSource=Input  idxRow=1  idxCol=1
      settings: SourceProductName=Raptor
  raptor_data_read3 : Raptor_lib/Data Storage/raptor_data_read  dataName='CMU2_FULLCHG_CAPACITY'  dataShape=Scalar  idxSource=Input  idxRow=1  idxCol=1
      settings: SourceProductName=Raptor
  raptor_data_read4 : Raptor_lib/Data Storage/raptor_data_read  dataName='CMU2_REMAIN_CAPACITY'  dataShape=Scalar  idxSource=Input  idxRow=1  idxCol=1
      settings: SourceProductName=Raptor
  raptor_data_read6 : Raptor_lib/Data Storage/raptor_data_read  dataName='CMU2_E3_ERR_CODE'  dataShape=Scalar  idxSource=Input  idxRow=1  idxCol=1
      settings: SourceProductName=Raptor
  wires:
  Fcn1/1 -> Data Type Conversion4/1
  Data Type Conversion5/1 -> raptor_can_txmsg/3
  Data Type Conversion4/1 -> raptor_can_txmsg/5
  raptor_data_read4/1 -> Data Type Conversion3/1
  Data Type Conversion3/1 -> raptor_can_txmsg/6
  raptor_data_read1/1 -> Fcn1/1
  Data Type Conversion1/1 -> raptor_can_txmsg/1
  Data Type Conversion2/1 -> raptor_can_txmsg/2
  raptor_data_read3/1 -> Data Type Conversion5/1
  Bitwise Operator/1 -> Shift Arithmetic1/1
  raptor_data_read2/1 -> raptor_can_txmsg/4
  Bitwise Operator1/1 -> Data Type Conversion/1
  raptor_data_read6/1 -> Bitwise Operator1/1, Bitwise Operator/1
  Shift Arithmetic1/1 -> Data Type Conversion1/1
  Data Type Conversion/1 -> Data Type Conversion2/1

== system EPT/Foreground_TimeBase_5ms/CAN/CAN2_exec/BCU vs ITRI//ARTC/Remote DAG2-5E7 ==
  Enable : EnablePort
  Trigger : TriggerPort  VariantControl=Variant  PortDimensions=1
  Data Type Conversion{1..4} (4 alike) : DataTypeConversion
  Fcn1 : Fcn  Expr=(u(1)-2)/0.01
  Fcn2 : Fcn  Expr=(u(1)-2)/0.01
  Fcn3 : Fcn  Expr=(u(1)+40)/0.5
  Fcn4 : Fcn  Expr=(u(1)+40)/0.5
  raptor_can_txmsg : Raptor_lib/CAN/raptor_can_txmsg  canDefinition=struct('dbcFile', 'BCUvsRMDA_CMU.dbc','message', 'RemoteDAG_5E7','comment', '','signals', {{'CMU2_Ibp','CMU2_Tcell_Max','CMU2_Tcell_Min','CMU2_Vbp','CMU2_Vcell_Max','CMU2_Vcell_Min'}},'enabled', [ 1 1 1 1 1 1;],'canBus', '''CAN2''','messageID', [ 1511;],'idMask', [ 536870911;],'payloadMask', [],'payloadValue', [],'period', [ 0;],'mailbox', '','queueSize', [ 1;],'label', [ 0;],'ver', [ 2;],'showID', [ 0;],'showRaw', [ 0;],'fill', [ 0;],'editID', [ 0;],'signalOrder', [ 1;])  canBus='CAN2'  queueSize=1  payloadMask=[]  payloadValue=[]  period=0  showID=0  label=0  idMask=hex2dec('1FFFFFFF')  fill=0  id=1511  showRaw=0  signalOrder=1  signalInfo={{struct('Name', 'CMU2_Ibp','Startbit', [ 0;],'SignalSize', [ 16;],'ByteOrder', 'BigEndian','ValueType', 'UNSIGNED','Class', 'uint16','Signed', [ 0;],'Factor', [ 0.02;],'Offset', [ -500;],'Min', [ 0;],'Max', [ 0;],'Units', '','Comment', '','StartBit', [ 8;]),struct('Name', 'CMU2_Vbp','Startbit', [ 0;],'SignalSize', [ 16;],'ByteOrder', 'BigEndian','ValueType', 'UNSIGNED','Class', 'uint16','Signed', [ 0;],'Factor', [ 0.01;],'Offset', [ 0;],'Min', [ 0;],'Max', [ 0;],'Units', '','Comment', '','StartBit', [ 24;]),struct('Name', 'CMU2_Vcell_Max','Startbit', [ 0;],'SignalSize', [ 8;],'ByteOrder', 'BigEndian','ValueType', 'UNSIGNED','Class', 'uint8','Signed', [ 0;],'Factor', [ 1;],'Offset', [ 0;],'Min', [ 0;],'Max', [ 0;],'Units', '','Comment', '','StartBit', [ 32;]),struct('Name', 'CMU2_Vcell_Min','Startbit', [ 0;],'SignalSize', [ 8;],'ByteOrder', 'BigEndian','ValueType', 'UNSIGNED','Class', 'uint8','Signed', [ 0;],'Factor', [ 1;],'Offset', [ 0;],'Min', [ 0;],'Max', [ 0;],'Units', '','Comment', '','StartBit', [ 40;]),struct('Name', 'CMU2_Tcell_Max','Startbit', [ 0;],'SignalSize', [ 8;],'ByteOrder', 'BigEndian','ValueType', 'UNSIGNED','Class', 'uint8','Signed', [ 0;],'Factor', [ 1;],'Offset', [ 0;],'Min', [ 0;],'Max', [ 0;],'Units', '','Comment', '','StartBit', [ 48;]),struct('Name', 'CMU2_Tcell_Min','Startbit', [ 0;],'SignalSize', [ 8;],'ByteOrder', 'BigEndian','ValueType', 'UNSIGNED','Class', 'uint8','Signed', [ 0;],'Factor', [ 1;],'Offset', [ 0;],'Min', [ 0;],'Max', [ 0;],'Units', '','Comment', '','StartBit', [ 56;])}}
      settings: SourceProductName=Raptor
  raptor_data_read : Raptor_lib/Data Storage/raptor_data_read  dataName='CMU2_CELL_VOLT_MAX'  dataShape=Scalar  idxSource=Input  idxRow=1  idxCol=1
      settings: SourceProductName=Raptor
  raptor_data_read1 : Raptor_lib/Data Storage/raptor_data_read  dataName='CMU2_CELL_VOLT_MIN'  dataShape=Scalar  idxSource=Input  idxRow=1  idxCol=1
      settings: SourceProductName=Raptor
  raptor_data_read2 : Raptor_lib/Data Storage/raptor_data_read  dataName='CMU2_CELL_TEMP_MIN'  dataShape=Scalar  idxSource=Input  idxRow=1  idxCol=1
      settings: SourceProductName=Raptor
  raptor_data_read3 : Raptor_lib/Data Storage/raptor_data_read  dataName='CMU2_BATT_CURR'  dataShape=Scalar  idxSource=Input  idxRow=1  idxCol=1
      settings: SourceProductName=Raptor
  raptor_data_read4 : Raptor_lib/Data Storage/raptor_data_read  dataName='CMU2_BATT_VOLT'  dataShape=Scalar  idxSource=Input  idxRow=1  idxCol=1
      settings: SourceProductName=Raptor
  raptor_data_read5 : Raptor_lib/Data Storage/raptor_data_read  dataName='CMU2_CELL_TEMP_MAX'  dataShape=Scalar  idxSource=Input  idxRow=1  idxCol=1
      settings: SourceProductName=Raptor
  wires:
  raptor_data_read2/1 -> Fcn4/1
  Data Type Conversion3/1 -> raptor_can_txmsg/3
  Fcn4/1 -> Data Type Conversion3/1
  raptor_data_read5/1 -> Fcn3/1
  Data Type Conversion2/1 -> raptor_can_txmsg/2
  Fcn3/1 -> Data Type Conversion2/1
  Data Type Conversion4/1 -> raptor_can_txmsg/6
  Data Type Conversion1/1 -> raptor_can_txmsg/5
  raptor_data_read/1 -> Fcn2/1
  Fcn2/1 -> Data Type Conversion1/1
  raptor_data_read1/1 -> Fcn1/1
  Fcn1/1 -> Data Type Conversion4/1
  raptor_data_read3/1 -> raptor_can_txmsg/1
  raptor_data_read4/1 -> raptor_can_txmsg/4

== system EPT/Foreground_TimeBase_5ms/CAN/CAN2_exec/BCU vs ITRI//ARTC/Remote DAG2-5E8 ==
  Enable : EnablePort
  Trigger : TriggerPort  VariantControl=Variant  PortDimensions=1
  Data Type Conversion{1..8} (8 alike) : DataTypeConversion
  Fcn{,1..7} (8 alike) : Fcn  Expr=(u(1)-2)/0.01
  raptor_can_txmsg : Raptor_lib/CAN/raptor_can_txmsg  canDefinition=struct('dbcFile', 'BCUvsRMDA_CMU.dbc','message', 'RemoteDAG_5E8','comment', '','signals', {{'CMU2_Vcell_V01','CMU2_Vcell_V02','CMU2_Vcell_V03','CMU2_Vcell_V04','CMU2_Vcell_V05','CMU2_Vcell_V06','CMU2_Vcell_V07','CMU2_Vcell_V08'}},'enabled', [ 1 1 1 1 1 1 1 1;],'canBus', '''CAN2''','messageID', [ 1512;],'idMask', [ 536870911;],'payloadMask', [],'payloadValue', [],'period', [ 0;],'mailbox', '','queueSize', [ 1;],'label', [ 0;],'ver', [ 2;],'showID', [ 0;],'showRaw', [ 0;],'fill', [ 0;],'editID', [ 0;],'signalOrder', [ 1;])  canBus='CAN2'  queueSize=1  payloadMask=[]  payloadValue=[]  period=0  showID=0  label=0  idMask=hex2dec('1FFFFFFF')  fill=0  id=1512  showRaw=0  signalOrder=1  signalInfo={{struct('Name', 'CMU2_Vcell_V01','Startbit', [ 0;],'SignalSize', [ 8;],'ByteOrder', 'BigEndian','ValueType', 'UNSIGNED','Class', 'uint8','Signed', [ 0;],'Factor', [ 1;],'Offset', [ 0;],'Min', [ 0;],'Max', [ 0;],'Units', '','Comment', '','StartBit', [ 0;]),struct('Name', 'CMU2_Vcell_V02','Startbit', [ 0;],'SignalSize', [ 8;],'ByteOrder', 'BigEndian','ValueType', 'UNSIGNED','Class', 'uint8','Signed', [ 0;],'Factor', [ 1;],'Offset', [ 0;],'Min', [ 0;],'Max', [ 0;],'Units', '','Comment', '','StartBit', [ 8;]),struct('Name', 'CMU2_Vcell_V03','Startbit', [ 0;],'SignalSize', [ 8;],'ByteOrder', 'BigEndian','ValueType', 'UNSIGNED','Class', 'uint8','Signed', [ 0;],'Factor', [ 1;],'Offset', [ 0;],'Min', [ 0;],'Max', [ 0;],'Units', '','Comment', '','StartBit', [ 16;]),struct('Name', 'CMU2_Vcell_V04','Startbit', [ 0;],'SignalSize', [ 8;],'ByteOrder', 'BigEndian','ValueType', 'UNSIGNED','Class', 'uint8','Signed', [ 0;],'Factor', [ 1;],'Offset', [ 0;],'Min', [ 0;],'Max', [ 0;],'Units', '','Comment', '','StartBit', [ 24;]),struct('Name', 'CMU2_Vcell_V05','Startbit', [ 0;],'SignalSize', [ 8;],'ByteOrder', 'BigEndian','ValueType', 'UNSIGNED','Class', 'uint8','Signed', [ 0;],'Factor', [ 1;],'Offset', [ 0;],'Min', [ 0;],'Max', [ 0;],'Units', '','Comment', '','StartBit', [ 32;]),struct('Name', 'CMU2_Vcell_V06','Startbit', [ 0;],'SignalSize', [ 8;],'ByteOrder', 'BigEndian','ValueType', 'UNSIGNED','Class', 'uint8','Signed', [ 0;],'Factor', [ 1;],'Offset', [ 0;],'Min', [ 0;],'Max', [ 0;],'Units', '','Comment', '','StartBit', [ 40;]),struct('Name', 'CMU2_Vcell_V07','Startbit', [ 0;],'SignalSize', [ 8;],'ByteOrder', 'BigEndian','ValueType', 'UNSIGNED','Class', 'uint8','Signed', [ 0;],'Factor', [ 1;],'Offset', [ 0;],'Min', [ 0;],'Max', [ 0;],'Units', '','Comment', '','StartBit', [ 48;]),struct('Name', 'CMU2_Vcell_V08','Startbit', [ 0;],'SignalSize', [ 8;],'ByteOrder', 'BigEndian','ValueType', 'UNSIGNED','Class', 'uint8','Signed', [ 0;],'Factor', [ 1;],'Offset', [ 0;],'Min', [ 0;],'Max', [ 0;],'Units', '','Comment', '','StartBit', [ 56;])}}
      settings: SourceProductName=Raptor
  raptor_data_read1 : Raptor_lib/Data Storage/raptor_data_read  dataName='CMU2_CELL02_VOLT'  dataShape=Scalar  idxSource=Input  idxRow=1  idxCol=1
      settings: SourceProductName=Raptor
  raptor_data_read2 : Raptor_lib/Data Storage/raptor_data_read  dataName='CMU2_CELL03_VOLT'  dataShape=Scalar  idxSource=Input  idxRow=1  idxCol=1
      settings: SourceProductName=Raptor
  raptor_data_read3 : Raptor_lib/Data Storage/raptor_data_read  dataName='CMU2_CELL01_VOLT'  dataShape=Scalar  idxSource=Input  idxRow=1  idxCol=1
      settings: SourceProductName=Raptor
  raptor_data_read4 : Raptor_lib/Data Storage/raptor_data_read  dataName='CMU2_CELL04_VOLT'  dataShape=Scalar  idxSource=Input  idxRow=1  idxCol=1
      settings: SourceProductName=Raptor
  raptor_data_read5 : Raptor_lib/Data Storage/raptor_data_read  dataName='CMU2_CELL05_VOLT'  dataShape=Scalar  idxSource=Input  idxRow=1  idxCol=1
      settings: SourceProductName=Raptor
  raptor_data_read6 : Raptor_lib/Data Storage/raptor_data_read  dataName='CMU2_CELL06_VOLT'  dataShape=Scalar  idxSource=Input  idxRow=1  idxCol=1
      settings: SourceProductName=Raptor
  raptor_data_read7 : Raptor_lib/Data Storage/raptor_data_read  dataName='CMU2_CELL07_VOLT'  dataShape=Scalar  idxSource=Input  idxRow=1  idxCol=1
      settings: SourceProductName=Raptor
  raptor_data_read8 : Raptor_lib/Data Storage/raptor_data_read  dataName='CMU2_CELL08_VOLT'  dataShape=Scalar  idxSource=Input  idxRow=1  idxCol=1
      settings: SourceProductName=Raptor
  wires:
  raptor_data_read8/1 -> Fcn7/1
  Fcn/1 -> Data Type Conversion4/1
  Fcn3/1 -> Data Type Conversion6/1
  Data Type Conversion3/1 -> raptor_can_txmsg/8
  Data Type Conversion5/1 -> raptor_can_txmsg/5
  Fcn5/1 -> Data Type Conversion1/1
  Fcn4/1 -> Data Type Conversion5/1
  Fcn6/1 -> Data Type Conversion2/1
  Fcn2/1 -> Data Type Conversion7/1
  raptor_data_read5/1 -> Fcn4/1
  Fcn7/1 -> Data Type Conversion3/1
  Fcn1/1 -> Data Type Conversion8/1
  raptor_data_read4/1 -> Fcn3/1
  Data Type Conversion1/1 -> raptor_can_txmsg/6
  Data Type Conversion2/1 -> raptor_can_txmsg/7
  Data Type Conversion4/1 -> raptor_can_txmsg/1
  Data Type Conversion8/1 -> raptor_can_txmsg/2
  Data Type Conversion7/1 -> raptor_can_txmsg/3
  Data Type Conversion6/1 -> raptor_can_txmsg/4
  raptor_data_read3/1 -> Fcn/1
  raptor_data_read1/1 -> Fcn1/1
  raptor_data_read6/1 -> Fcn5/1
  raptor_data_read2/1 -> Fcn2/1
  raptor_data_read7/1 -> Fcn6/1

== system EPT/Foreground_TimeBase_5ms/CAN/CAN2_exec/BCU vs ITRI//ARTC/Remote DAG2-5E9 ==
  Enable : EnablePort
  Trigger : TriggerPort  VariantControl=Variant  PortDimensions=1
  Data Type Conversion{1..8} (8 alike) : DataTypeConversion
  Fcn{,1..7} (8 alike) : Fcn  Expr=(u(1)-2)/0.01
  raptor_can_txmsg : Raptor_lib/CAN/raptor_can_txmsg  canDefinition=struct('dbcFile', 'BCUvsRMDA_CMU.dbc','message', 'RemoteDAG_5E9','comment', '','signals', {{'CMU2_Vcell_V09','CMU2_Vcell_V10','CMU2_Vcell_V11','CMU2_Vcell_V12','CMU2_Vcell_V13','CMU2_Vcell_V14','CMU2_Vcell_V15','CMU2_Vcell_V16'}},'enabled', [ 1 1 1 1 1 1 1 1;],'canBus', '''CAN2''','messageID', [ 1513;],'idMask', [ 536870911;],'payloadMask', [],'payloadValue', [],'period', [ 0;],'mailbox', '','queueSize', [ 1;],'label', [ 0;],'ver', [ 2;],'showID', [ 0;],'showRaw', [ 0;],'fill', [ 0;],'editID', [ 0;],'signalOrder', [ 1;])  canBus='CAN2'  queueSize=1  payloadMask=[]  payloadValue=[]  period=0  showID=0  label=0  idMask=hex2dec('1FFFFFFF')  fill=0  id=1513  showRaw=0  signalOrder=1  signalInfo={{struct('Name', 'CMU2_Vcell_V09','Startbit', [ 0;],'SignalSize', [ 8;],'ByteOrder', 'BigEndian','ValueType', 'UNSIGNED','Class', 'uint8','Signed', [ 0;],'Factor', [ 1;],'Offset', [ 0;],'Min', [ 0;],'Max', [ 0;],'Units', '','Comment', '','StartBit', [ 0;]),struct('Name', 'CMU2_Vcell_V10','Startbit', [ 0;],'SignalSize', [ 8;],'ByteOrder', 'BigEndian','ValueType', 'UNSIGNED','Class', 'uint8','Signed', [ 0;],'Factor', [ 1;],'Offset', [ 0;],'Min', [ 0;],'Max', [ 0;],'Units', '','Comment', '','StartBit', [ 8;]),struct('Name', 'CMU2_Vcell_V11','Startbit', [ 0;],'SignalSize', [ 8;],'ByteOrder', 'BigEndian','ValueType', 'UNSIGNED','Class', 'uint8','Signed', [ 0;],'Factor', [ 1;],'Offset', [ 0;],'Min', [ 0;],'Max', [ 0;],'Units', '','Comment', '','StartBit', [ 16;]),struct('Name', 'CMU2_Vcell_V12','Startbit', [ 0;],'SignalSize', [ 8;],'ByteOrder', 'BigEndian','ValueType', 'UNSIGNED','Class', 'uint8','Signed', [ 0;],'Factor', [ 1;],'Offset', [ 0;],'Min', [ 0;],'Max', [ 0;],'Units', '','Comment', '','StartBit', [ 24;]),struct('Name', 'CMU2_Vcell_V13','Startbit', [ 0;],'SignalSize', [ 8;],'ByteOrder', 'BigEndian','ValueType', 'UNSIGNED','Class', 'uint8','Signed', [ 0;],'Factor', [ 1;],'Offset', [ 0;],'Min', [ 0;],'Max', [ 0;],'Units', '','Comment', '','StartBit', [ 32;]),struct('Name', 'CMU2_Vcell_V14','Startbit', [ 0;],'SignalSize', [ 8;],'ByteOrder', 'BigEndian','ValueType', 'UNSIGNED','Class', 'uint8','Signed', [ 0;],'Factor', [ 1;],'Offset', [ 0;],'Min', [ 0;],'Max', [ 0;],'Units', '','Comment', '','StartBit', [ 40;]),struct('Name', 'CMU2_Vcell_V15','Startbit', [ 0;],'SignalSize', [ 8;],'ByteOrder', 'BigEndian','ValueType', 'UNSIGNED','Class', 'uint8','Signed', [ 0;],'Factor', [ 1;],'Offset', [ 0;],'Min', [ 0;],'Max', [ 0;],'Units', '','Comment', '','StartBit', [ 48;]),struct('Name', 'CMU2_Vcell_V16','Startbit', [ 0;],'SignalSize', [ 8;],'ByteOrder', 'BigEndian','ValueType', 'UNSIGNED','Class', 'uint8','Signed', [ 0;],'Factor', [ 1;],'Offset', [ 0;],'Min', [ 0;],'Max', [ 0;],'Units', '','Comment', '','StartBit', [ 56;])}}
      settings: SourceProductName=Raptor
  raptor_data_read1 : Raptor_lib/Data Storage/raptor_data_read  dataName='CMU2_CELL10_VOLT'  dataShape=Scalar  idxSource=Input  idxRow=1  idxCol=1
      settings: SourceProductName=Raptor
  raptor_data_read2 : Raptor_lib/Data Storage/raptor_data_read  dataName='CMU2_CELL11_VOLT'  dataShape=Scalar  idxSource=Input  idxRow=1  idxCol=1
      settings: SourceProductName=Raptor
  raptor_data_read3 : Raptor_lib/Data Storage/raptor_data_read  dataName='CMU2_CELL09_VOLT'  dataShape=Scalar  idxSource=Input  idxRow=1  idxCol=1
      settings: SourceProductName=Raptor
  raptor_data_read4 : Raptor_lib/Data Storage/raptor_data_read  dataName='CMU2_CELL12_VOLT'  dataShape=Scalar  idxSource=Input  idxRow=1  idxCol=1
      settings: SourceProductName=Raptor
  raptor_data_read5 : Raptor_lib/Data Storage/raptor_data_read  dataName='CMU2_CELL13_VOLT'  dataShape=Scalar  idxSource=Input  idxRow=1  idxCol=1
      settings: SourceProductName=Raptor
  raptor_data_read6 : Raptor_lib/Data Storage/raptor_data_read  dataName='CMU2_CELL14_VOLT'  dataShape=Scalar  idxSource=Input  idxRow=1  idxCol=1
      settings: SourceProductName=Raptor
  raptor_data_read7 : Raptor_lib/Data Storage/raptor_data_read  dataName='CMU2_CELL15_VOLT'  dataShape=Scalar  idxSource=Input  idxRow=1  idxCol=1
      settings: SourceProductName=Raptor
  raptor_data_read8 : Raptor_lib/Data Storage/raptor_data_read  dataName='CMU2_CELL16_VOLT'  dataShape=Scalar  idxSource=Input  idxRow=1  idxCol=1
      settings: SourceProductName=Raptor
  wires:
  Data Type Conversion4/1 -> raptor_can_txmsg/1
  Data Type Conversion8/1 -> raptor_can_txmsg/2
  Data Type Conversion7/1 -> raptor_can_txmsg/3
  Data Type Conversion6/1 -> raptor_can_txmsg/4
  Data Type Conversion5/1 -> raptor_can_txmsg/5
  Data Type Conversion1/1 -> raptor_can_txmsg/6
  Data Type Conversion2/1 -> raptor_can_txmsg/7
  raptor_data_read1/1 -> Fcn1/1
  Fcn7/1 -> Data Type Conversion3/1
  raptor_data_read5/1 -> Fcn4/1
  Fcn2/1 -> Data Type Conversion7/1
  Fcn1/1 -> Data Type Conversion8/1
  raptor_data_read4/1 -> Fcn3/1
  Fcn/1 -> Data Type Conversion4/1
  Fcn4/1 -> Data Type Conversion5/1
  raptor_data_read7/1 -> Fcn6/1
  raptor_data_read2/1 -> Fcn2/1
  raptor_data_read6/1 -> Fcn5/1
  Fcn3/1 -> Data Type Conversion6/1
  Fcn6/1 -> Data Type Conversion2/1
  Fcn5/1 -> Data Type Conversion1/1
  raptor_data_read3/1 -> Fcn/1
  raptor_data_read8/1 -> Fcn7/1
  Data Type Conversion3/1 -> raptor_can_txmsg/8
